simulink model "line_follower"  (R2021a)
settings: Solver=VariableStepAuto  StartTime=0.0  StopTime=40  RelTol=1e-3
undefined symbols (not defined in the file): gray
libraries: vrlib x3, visiontextngfix x2, dspvision x1, visionconversions x1, deeplib x1, pid_lib x1, robotmobilelib x1
settings Model: EnablePacing=on  Creator=tkikawad  LastModifiedBy=tkikawad
settings SolverCC: AlgebraicLoopSolver=TrustRegion
settings DebuggingCC: SFMachineParentedDataDiag=warning
settings SFSimCC: SimTargetLang=C++  SimDLAutoTuning=off

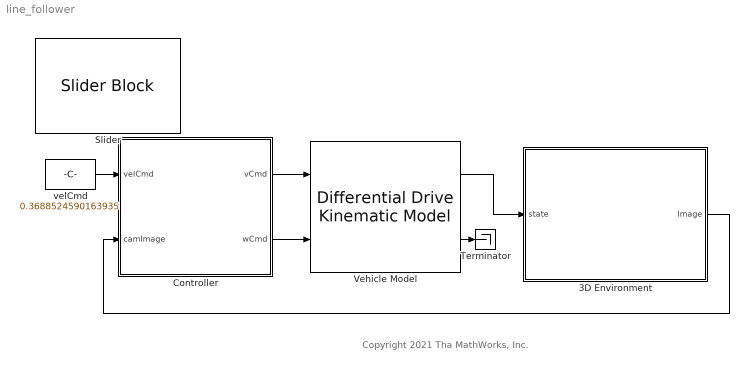
== system line_follower ==
  note: Copyright 2021 Tha MathWorks, Inc.
  3D Environment : Subsystem  mask{world=World1, z=0}
      mask prompts: world "Select World:"
      mask init:
      | switch world
      |   case 1
      |     z = 0;
      |     imgfile =  'course.png';
      |   case 2
      |     z = 10;
      |     imgfile =  'course_circle.png';
      |   case 3
      |     z = 20;
      |     imgfile =  'course_curve.png';
      |   otherwise
      |     imgfile =  'course.png';
      | end
      | assignin('base','world',world)
      mask TypeOptions world: World1 | World2 | World3
      mask DialogControl DescGroupVar Prompt: 3D Environment
      mask DialogControl DescTextVar Prompt: 3D environment using Simulink 3D Animation.
      mask Display:
      | image(imgfile,[0.15 0.15 0.7 0.7]);
      | text(0.5, 0.1, "World" + world,...
      |     'horizontalAlignment', 'center',...
      |     'verticalAlignment', 'top');
  Controller : Subsystem
  Slider : SliderBlock  ScaleMax=1
  Terminator : Terminator
  Vehicle Model : robotmobilelib/Differential Drive Kinematic Model  VehicleInputs=Vehicle Speed & Heading Angular Velocity  WheelRadius=0.03  WheelSpeedRange=[-2*pi*5 2*pi*5]  TrackWidth=0.1  InitialState="[0.375, 0,  pi/2]"  SimulateUsing=Interpreted execution
      settings: SourceProductBaseCode=RO
  velCmd : Constant  Value=0.3688524590163935  SampleTime=-1
  wires:
  3D Environment/1(Image) -> Controller/2(camImage)
  velCmd/1 -> Controller/1(velCmd)
  Vehicle Model/1 -> 3D Environment/1(state)
  Controller/1(vCmd) -> Vehicle Model/1
  Controller/2(wCmd) -> Vehicle Model/2
  Vehicle Model/2 -> Terminator/1

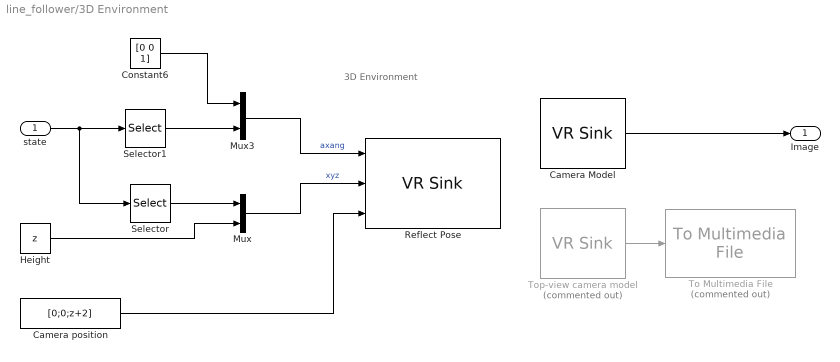
== system line_follower/3D Environment ==
  note: 3D Environment
  state : Inport
  Camera Model : vrlib/VR Sink  InstantiateOnLoad=on  SampleTime=0.1  ViewEnable=on  RemoteChange=off  RemoteView=off  WorldFileName=robotTrainWorld.wrl  AutoView=off  VideoDimensions=[180,320]  AllowVariableSize=off  FigureProperties="{'Position', 'Name', 'Viewpoint', 'CameraBound', 'CameraDirection', 'CameraPosition', 'CameraUpVector', 'ZoomFactor', 'Antialiasing', 'Headlight', 'Lighting', 'NavPanel', 'Sound', 'StatusBar', 'Stereo3D', 'Stereo3DCameraOffset', 'Stereo3DHIT', 'ToolBar', 'Textures', 'Transparency', 'Triad', 'Wireframe', 'NavZones', 'NavMode', 'NavSpeed', 'CaptureFileFormat', 'CaptureFileName', 'Record2DCompressMethod', 'Record2DCompressQuality', 'Record2D', 'Record2DFileName', 'Record2DFPS'; [5.0000000000000000e+00   6.0000000000000000e+01   3.2000000000000000e+02   1.8000000000000000e+02], '', '_untitled_1', 'on', [0.0000000000000000e+00   0.0000000000000000e+00  -1.0000000000000000e+00], [0.0000000000000000e+00   0.0000000000000000e+00   0.0000000000000000e+00], [0.0000000000000000e+00   1.0000000000000000e+00   0.0000000000000000e+00], [1.0000000000000000e+00], 'off', 'on', 'on', 'none', 'on', 'off', 'off', [1.0000000149011612e-01], [0.0000000000000000e+00], 'off', 'on', 'on', 'none', 'off', 'off', 'fly', 'normal', 'tif', '%f_anim_%n.tif', 'auto', [7.5000000000000000e+01], 'off', '***video***', 'auto'}"
  Camera position : Constant  Value=[0;0;z+2]
  Constant6 : Constant  Value=[0 0 1]
  Height : Constant  Value=z
  Mux : Mux  Inputs=2
  Mux3 : Mux  Inputs=2
  Reflect Pose : vrlib/VR Sink  InstantiateOnLoad=on  SampleTime=0.01  ViewEnable=on  RemoteChange=off  RemoteView=off  FieldsWritten=robot.rotation.4.1.1.double#robot.translation.3.1.1.double#worldCamera.position.3.1.1.double  WorldFileName=robotTrainWorld.wrl  AutoView=on  VideoDimensions=[]  AllowVariableSize=off  FigureProperties="{'Position', 'Name', 'Viewpoint', 'CameraBound', 'CameraDirection', 'CameraPosition', 'CameraUpVector', 'ZoomFactor', 'Antialiasing', 'Headlight', 'Lighting', 'NavPanel', 'Sound', 'StatusBar', 'Stereo3D', 'Stereo3DCameraOffset', 'Stereo3DHIT', 'ToolBar', 'Textures', 'Transparency', 'Triad', 'Wireframe', 'NavZones', 'NavMode', 'NavSpeed', 'CaptureFileFormat', 'CaptureFileName', 'Record2DCompressMethod', 'Record2DCompressQuality', 'Record2D', 'Record2DFileName', 'Record2DFPS'; [-4.5100000000000000e+02   4.3700000000000000e+02   4.5100000000000000e+02   2.3100000000000000e+02], '', '_untitled_2', 'on', [0.0000000000000000e+00   0.0000000000000000e+00  -1.0000000000000000e+00], [0.0000000000000000e+00   0.0000000000000000e+00   0.0000000000000000e+00], [0.0000000000000000e+00   1.0000000000000000e+00   0.0000000000000000e+00], [1.4641000000000006e+00], 'off', 'on', 'on', 'halfbar', 'on', 'on', 'off', [1.0000000149011612e-01], [0.0000000000000000e+00], 'on', 'on', 'on', 'none', 'off', 'off', 'fly', 'normal', 'tif', '%f_anim_%n.tif', 'auto', [7.5000000000000000e+01], 'off', '%f_anim_%n.avi', 'auto'}"
  Selector : Selector  InputPortWidth=3  IndexOptions=Index vector (dialog)  Indices=[1 2]  OutputSizes=1
  Selector1 : Selector  InputPortWidth=3  IndexOptions=Index vector (dialog)  Indices=3  OutputSizes=1
  To Multimedia File : dspvision/To Multimedia File  Commented=on  outputFilename=topview.mp4  streamSelection=Video only  videoCompressor=None (uncompressed)  audioCompressor=None (uncompressed)  imagePorts=One multidimensional signal  fileType=MPEG4  audioDatatype=Determine from input data type  fourcc=RGB  videoQuality=75  mj2000CompFactor=10
  Top-view camera model : vrlib/VR Sink  Commented=on  InstantiateOnLoad=on  SampleTime=1/30  ViewEnable=on  RemoteChange=off  RemoteView=off  WorldFileName=robotTrainWorld.wrl  AutoView=off  VideoDimensions=[480,640]  AllowVariableSize=off  FigureProperties="{'Position', 'Name', 'Viewpoint', 'CameraBound', 'CameraDirection', 'CameraPosition', 'CameraUpVector', 'ZoomFactor', 'Antialiasing', 'Headlight', 'Lighting', 'NavPanel', 'Sound', 'StatusBar', 'Stereo3D', 'Stereo3DCameraOffset', 'Stereo3DHIT', 'ToolBar', 'Textures', 'Transparency', 'Triad', 'Wireframe', 'NavZones', 'NavMode', 'NavSpeed', 'CaptureFileFormat', 'CaptureFileName', 'Record2DCompressMethod', 'Record2DCompressQuality', 'Record2D', 'Record2DFileName', 'Record2DFPS'; [9.6600000000000000e+02   6.0000000000000000e+01   6.4000000000000000e+02   4.8000000000000000e+02], '', '_untitled_2', 'on', [0.0000000000000000e+00   0.0000000000000000e+00  -1.0000000000000000e+00], [0.0000000000000000e+00   0.0000000000000000e+00   0.0000000000000000e+00], [0.0000000000000000e+00   1.0000000000000000e+00   0.0000000000000000e+00], [1.0000000000000000e+00], 'on', 'on', 'on', 'none', 'on', 'off', 'off', [1.0000000149011612e-01], [0.0000000000000000e+00], 'off', 'on', 'on', 'none', 'off', 'off', 'fly', 'normal', 'tif', '%f_anim_%n.tif', 'auto', [7.5000000000000000e+01], 'off', '***video***', 'auto'}"
  Image : Outport
  wires:
  Selector/1 -> Mux/1
  Camera position/1 -> Reflect Pose/3
  Selector1/1 -> Mux3/2
  Mux3/1 -> Reflect Pose/1  "axang"
  state/1 -> Selector/1, Selector1/1
  Constant6/1 -> Mux3/1
  Mux/1 -> Reflect Pose/2  "xyz"
  Height/1 -> Mux/2
  Camera Model/1 -> Image/1
  Top-view camera model/1 -> To Multimedia File/1

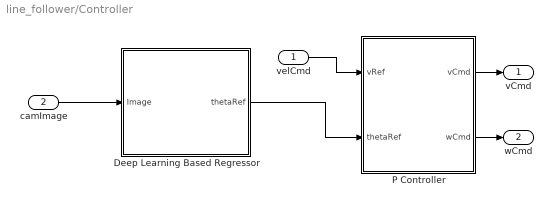
== system line_follower/Controller ==
  velCmd : Inport
  camImage : Inport  Port=2
  Deep Learning Based Regressor : Subsystem
  P Controller : Subsystem
  vCmd : Outport
  wCmd : Outport  Port=2
  wires:
  P Controller/2(wCmd) -> wCmd/1
  Deep Learning Based Regressor/1(thetaRef) -> P Controller/2(thetaRef)
  velCmd/1 -> P Controller/1(vRef)
  P Controller/1(vCmd) -> vCmd/1
  camImage/1 -> Deep Learning Based Regressor/1(Image)

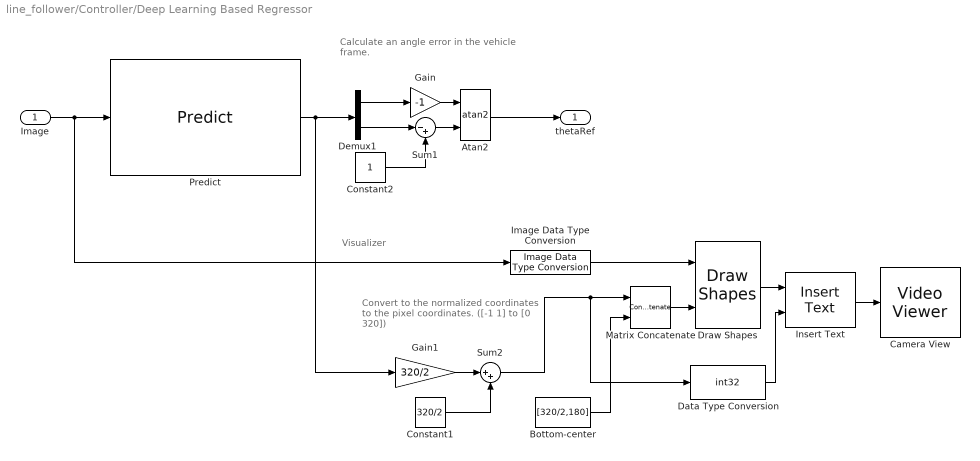
== system line_follower/Controller/Deep Learning Based Regressor ==
  note: Visualizer
  note: Calculate an angle error
      | in the vehicle frame.
  note: Convert to the normalized
      | coordinates to
      | the pixel coordinates.
      | ([-1 1] to [0 320])
  Image : Inport
  Atan2 : Trigonometry  Operator=atan2
  Bottom-center : Constant  Value=[320/2,180]  VectorParams1D=off
  Camera View : VideoViewer  colormapValue=gray(256)  FigPos=[-460 350 460 294]
  Constant1 : Constant  Value=320/2
  Constant2 : Constant  OutDataTypeStr=single
  Data Type Conversion : DataTypeConversion  OutDataTypeStr=int32
  Demux1 : Demux  Outputs=2
  Draw Shapes : visiontextngfix/Draw Shapes  shape=Lines  fill=off  lineWidth=3  fillClrSource=Specify via dialog  display=User-specified value  intensity=200  color=[1,0,0]  opacity=0.6  viewport=Entire image  antialiasing=on  inType=Obsolete  imagePorts=One multidimensional signal  roundingMode=Floor  overflowMode=off  memoryMode=Specify word length  memoryWordLength=16  prodOutputMode=Binary point scaling  prodOutputWordLength=32  prodOutputFracLength=14  memoryFracLength=15
  Gain : Gain  Gain=-1
  Gain1 : Gain  Gain=320/2
  Image Data Type Conversion : visionconversions/Image Data Type Conversion  outDT=single  isSigned=on  wordLen=16  numFracBits=0
      settings: SourceProductBaseCode=VP
  Insert Text : visiontextngfix/Insert Text  inputType=Obsolete  theText="'  Predicted point'"  getTextLocFrom=Input port  textLoc=[1 1]  getTextColorFrom=Specify via dialog  textColor=[1 0 0]  getTextIntensityFrom=Specify via dialog  textIntensity=0  getTextOpacityFrom=Specify via dialog  textOpacity=1.0  dummyVar2=0  dummyVar3=0  dummyVar4=0  imagePorts=One multidimensional signal  isInputTransposed=off  fontFace=LucidaSansRegular  dummyVar1=0  blockFontSize=12  antiAliased=on
      settings: SourceProductBaseCode=VP
  Matrix Concatenate : Concatenate  Mode=Multidimensional array  ConcatenateDimension=2
  Predict : deeplib/Predict  Network=Network from MAT-file  NetworkFunction=squeezenet  NetworkFilePath=mynet_new.mat  MiniBatchSize=1  InputDataFormats={ '', '' }  Predictions=on  Activations={}  ForceInterpretedSim=off  EnableDLNetwork=off
      settings: SourceProductBaseCode=NN
  Sum1 : Sum  Inputs=|-+
  Sum2 : Sum  Inputs=|++
  thetaRef : Outport
  wires:
  Demux1/1 -> Gain/1
  Atan2/1 -> thetaRef/1
  Demux1/2 -> Sum1/1
  Sum1/1 -> Atan2/2
  Constant2/1 -> Sum1/2
  Gain1/1 -> Sum2/1
  Sum2/1 -> Data Type Conversion/1, Matrix Concatenate/1
  Constant1/1 -> Sum2/2
  Predict/1 -> Gain1/1, Demux1/1
  Image/1 -> Predict/1, Image Data Type Conversion/1
  Draw Shapes/1 -> Insert Text/1
  Image Data Type Conversion/1 -> Draw Shapes/1
  Matrix Concatenate/1 -> Draw Shapes/2
  Bottom-center/1 -> Matrix Concatenate/2
  Insert Text/1 -> Camera View/1
  Data Type Conversion/1 -> Insert Text/2
  Gain/1 -> Atan2/1

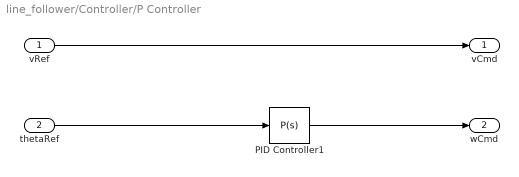
== system line_follower/Controller/P Controller ==
  vRef : Inport
  thetaRef : Inport  Port=2
  PID Controller1 : pid_lib/PID Controller  Controller=P  Form=Parallel  TimeDomain=Continuous-time  UseExternalTs=off  SampleTime=0.01  IntegratorMethod=Forward Euler  FilterMethod=Forward Euler  ControllerParametersSource=internal  P=1.5  I=0.01  D=0.5  UseFilter=on  N=100  TunerSelectOption=Transfer Function Based (PID Tuner App)  InitialConditionSource=internal  InitialConditionForIntegrator=0  InitialConditionForFilter=0  DifferentiatorICPrevScaledInput=0  ExternalReset=none  TrackingMode=off  Kt=1  LimitOutput=off  SatLimitsSource=internal  UpperSaturationLimit=inf  LowerSaturationLimit=-inf  LinearizeAsGain=on  AntiWindupMode=none  Kb=1  POutMin=[]  POutMax=[]  IOutMin=[]  IOutMax=[]  DOutMin=[]  DOutMax=[]  NOutMin=[]  NOutMax=[]  SumOutMin=[]  SumOutMax=[]  SaturationOutMin=[]  SaturationOutMax=[]  PParamMin=[]  PParamMax=[]  IParamMin=[]  IParamMax=[]  DParamMin=[]  DParamMax=[]  NParamMin=[]  NParamMax=[]  KbParamMin=[]  KbParamMax=[]  KtParamMin=[]  KtParamMax=[]  KbOutMin=[]  KbOutMax=[]  KtOutMin=[]  KtOutMax=[]  IntegratorOutMin=[]  IntegratorOutMax=[]  FilterOutMin=[]  FilterOutMax=[]  SumI1OutMin=[]  SumI1OutMax=[]  SumI2OutMin=[]  SumI2OutMax=[]  SumI3OutMin=[]  SumI3OutMax=[]  SumI4OutMin=[]  SumI4OutMax=[]  SumDOutMin=[]  SumDOutMax=[]  DifferentiatorOutMin=[]  DifferentiatorOutMax=[]  FilterDiffOutCoefMin=[]  FilterDiffOutCoefMax=[]  ReciprocalOutMin=[]  ReciprocalOutMax=[]  SumDenOutMin=[]  SumDenOutMax=[]  SumNumOutMin=[]  SumNumOutMax=[]  DivideOutMin=[]  DivideOutMax=[]  UdiffTsProdOutMin=[]  UdiffTsProdOutMax=[]  NTsProdOutMin=[]  NTsProdOutMax=[]  UintegralTsProdOutMin=[]  UintegralTsProdOutMax=[]  UngainTsProdOutMin=[]  UngainTsProdOutMax=[]  IntegratorContinuousStateAttributes=''  IntegratorStateMustResolveToSignalObject=off  IntegratorRTWStateStorageClass=Auto  FilterContinuousStateAttributes=''  FilterStateMustResolveToSignalObject=off  FilterRTWStateStorageClass=Auto  ParallelPVariant=InternalParameters  IdealPVariant=Disabled  IVariant=Disabled  DVariant=Disabled  IntegratorVariant=Disabled  SatVariant=Disabled  AWVariant=Disabled  PCopyVariant=Disabled  TRVariant=Disabled  FdbkBlocksVariant=Forward  IdealPFdbkVariant=Disabled  SatFdbkVariant=Disabled  DerivativeFilterVariant=Disabled  NVariant=Disabled  NCopyVariant=Disabled_SignalSpec  FilterICVariant=Disabled  IntegratorICVariant=Disabled  ExternalResetVariant=Disabled  TRSumVariant=Passthrough  SumFdbkVariant=Disabled  SumVariant=Passthrough_P  TsampFilterVariant=InternalTs  TsampNgainVariant=Passthrough  TsampIntegralVariant=Disabled_SignalSpec  ExternalSaturationOutDataTypeStr=Inherit: Same as second input
  vCmd : Outport
  wCmd : Outport  Port=2
  wires:
  vRef/1 -> vCmd/1
  PID Controller1/1 -> wCmd/1
  thetaRef/1 -> PID Controller1/1
